simulink model "a2messy2"  (R2014b)
settings: Solver=ode45  StartTime=0.0  StopTime=1000  RelTol=1e-7
values from neighbouring files (symbols this model uses):
  g1 = 10    [a2messym.m]
  g2 = 10    [a2messym.m]
  g3 = 10    [a2messym.m]
  g4 = 10    [a2messym.m]
settings Model: Creator=zhouy  LastModifiedBy=zhouy

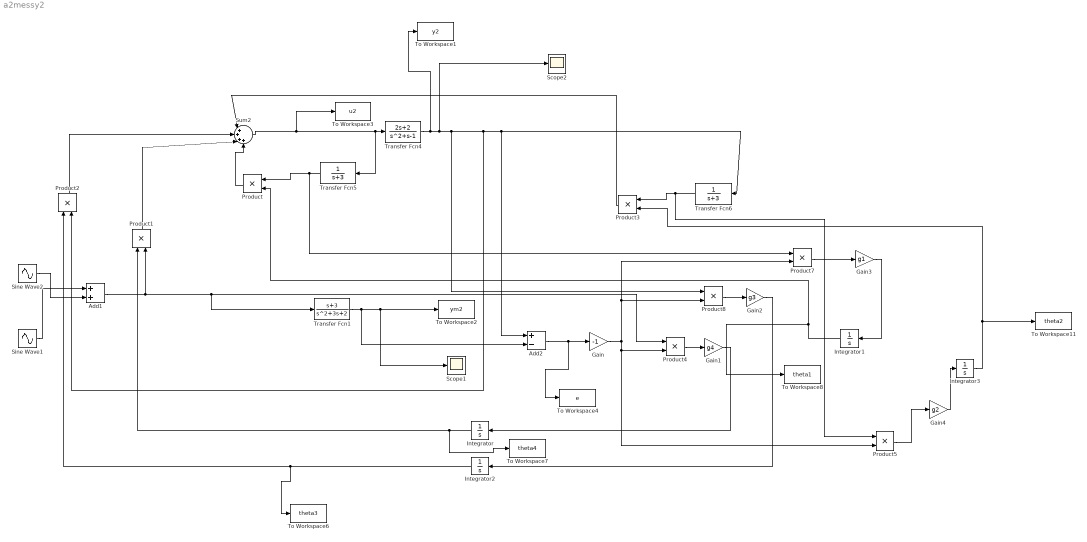
== system a2messy2 ==
  Add1 : Sum
  Add2 : Sum  Inputs=+-
  Gain : Gain  Gain=-1
  Gain1 : Gain  Gain=g4
  Gain2 : Gain  Gain=g3
  Gain3 : Gain  Gain=g1
  Gain4 : Gain  Gain=g2
  Integrator : Integrator
  Integrator1 : Integrator  InitialCondition=1.5
  Integrator2 : Integrator  InitialCondition=-1.5
  Integrator3 : Integrator  InitialCondition=2
  Product{,1..5,7..8} (8 alike) : Product
  Scope1 : Scope
  Scope2 : Scope
  Sine Wave1 : Sin  Frequency=3  SampleTime=0
  Sine Wave2 : Sin  SampleTime=0
  Sum2 : Sum  Inputs=|++++
  To Workspace1 : ToWorkspace  VariableName=y2  SaveFormat=Timeseries  SampleTime=-1
  To Workspace11 : ToWorkspace  VariableName=theta2  SaveFormat=Timeseries  SampleTime=-1
  To Workspace2 : ToWorkspace  VariableName=ym2  SaveFormat=Timeseries  SampleTime=-1
  To Workspace3 : ToWorkspace  VariableName=u2  SaveFormat=Timeseries  SampleTime=-1
  To Workspace4 : ToWorkspace  VariableName=e  SaveFormat=Timeseries  SampleTime=-1
  To Workspace6 : ToWorkspace  VariableName=theta3  SaveFormat=Timeseries  SampleTime=-1
  To Workspace7 : ToWorkspace  VariableName=theta4  SaveFormat=Timeseries  SampleTime=-1
  To Workspace8 : ToWorkspace  VariableName=theta1  SaveFormat=Timeseries  SampleTime=-1
  Transfer Fcn1 : TransferFcn  Numerator=[1 3]  Denominator=[1 3 2]
  Transfer Fcn4 : TransferFcn  Numerator=[2 2]  Denominator=[1 1 -1]
  Transfer Fcn5 : TransferFcn  Denominator=[1 3]
  Transfer Fcn6 : TransferFcn  Denominator=[1 3]
  wires:
  Add1/1 -> Product4/1, Transfer Fcn1/1, Product1/2
  Transfer Fcn1/1 -> Add2/2, Scope1/1, To Workspace2/1
  Sum2/1 -> To Workspace3/1, Transfer Fcn5/1, Transfer Fcn4/1
  Transfer Fcn5/1 -> Product7/1, Product/1
  Product/1 -> Sum2/4
  Product1/1 -> Sum2/3
  Product2/1 -> Sum2/2
  Transfer Fcn4/1 -> To Workspace1/1, Scope2/1, Product8/1, Product2/2, Add2/1, Transfer Fcn6/1
  Transfer Fcn6/1 -> Product5/1, Product3/1
  Product3/1 -> Sum2/1
  Gain/1 -> Product7/2, Product8/2, Product5/2, Product4/2
  Product4/1 -> Gain1/1
  Gain1/1 -> Integrator/1
  Integrator/1 -> To Workspace7/1, Product1/1
  Product8/1 -> Gain2/1
  Product7/1 -> Gain3/1
  Gain3/1 -> Integrator1/1
  Integrator1/1 -> To Workspace8/1, Product/2
  Integrator2/1 -> To Workspace6/1, Product2/1
  Product5/1 -> Gain4/1
  Gain4/1 -> Integrator3/1
  Integrator3/1 -> To Workspace11/1, Product3/2
  Sine Wave2/1 -> Add1/2
  Sine Wave1/1 -> Add1/1
  Add2/1 -> To Workspace4/1, Gain/1
  Gain2/1 -> Integrator2/1
